simulink model "equation"  (R2020b)
settings: Solver=FixedStepDiscrete  StartTime=0.0  StopTime=10.0  FixedStep=1  RelTol=1e-3
settings Model: Creator=Aradhana desai  LastModifiedBy=Aradhana desai

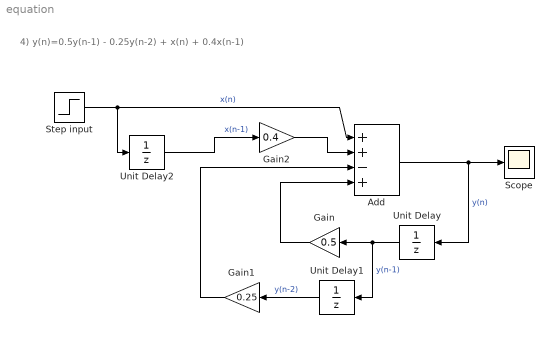
== system equation ==
  note: 4) y(n)=0.5y(n-1) - 0.25y(n-2) + x(n) + 0.4x(n-1)
  Add : Sum  Inputs=++-+
  Gain : Gain  Gain=0.5
  Gain1 : Gain  Gain=0.25
  Gain2 : Gain  Gain=0.4
  Scope : Scope
  Step input : Step  SampleTime=0
  Unit Delay : UnitDelay  SampleTime=-1  HasFrameUpgradeWarning=on
  Unit Delay1 : UnitDelay  SampleTime=-1  HasFrameUpgradeWarning=on
  Unit Delay2 : UnitDelay  SampleTime=-1  HasFrameUpgradeWarning=on
  wires:
  Add/1 -> Unit Delay/1, Scope/1  "y(n)"
  Unit Delay/1 -> Unit Delay1/1, Gain/1  "y(n-1)"
  Gain/1 -> Add/4
  Unit Delay1/1 -> Gain1/1  "y(n-2)"
  Gain1/1 -> Add/3
  Unit Delay2/1 -> Gain2/1  "x(n-1)"
  Gain2/1 -> Add/2
  Step input/1 -> Unit Delay2/1, Add/1  "x(n)"
